simulink model "LQR_controller_V2"  (R2023b)
settings: Solver=VariableStepAuto  StartTime=0.0  StopTime=10.0  RelTol=1e-3
undefined symbols (not defined in the file): A_obs, B_obs, C_obs, K_f_lqr, K_lqr, L
libraries: cstblocks x1
settings Model: Creator=torb  LastModifiedBy=torb

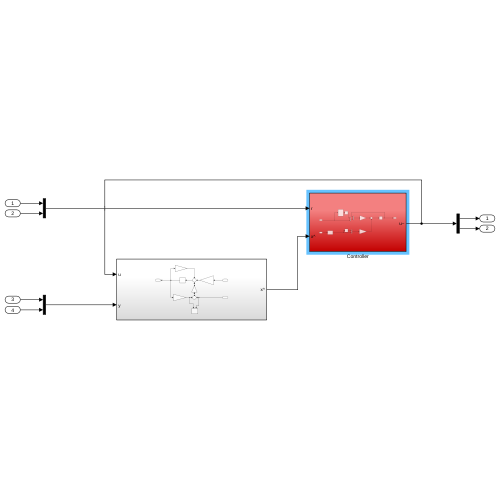
[thumbnail: Simulink's stored preview of the top-level diagram]
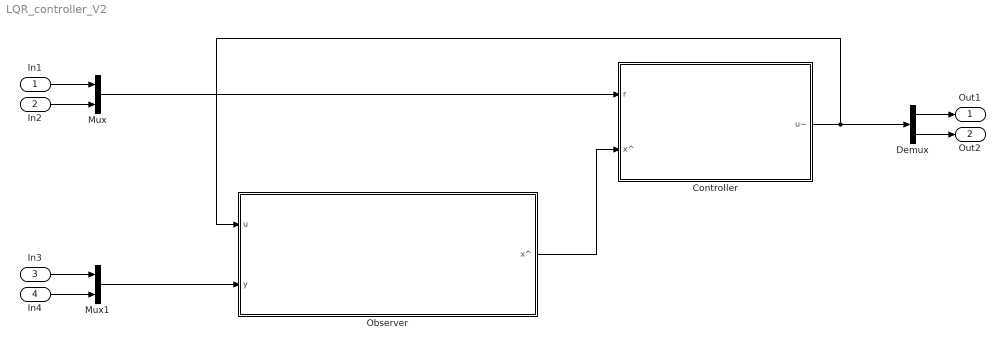
== system LQR_controller_V2 ==
  In1 : Inport
  In2 : Inport  Port=2
  In3 : Inport  Port=3
  In4 : Inport  Port=4
  Controller : Subsystem
  Demux : Demux  Outputs=2
  Mux : Mux  Inputs=2
  Mux1 : Mux  Inputs=2
  Observer : Subsystem
  Out1 : Outport
  Out2 : Outport  Port=2
  wires:
  Mux/1 -> Controller/1(r)
  Controller/1(u~) -> Demux/1, Observer/1(u)
  Observer/1(x^) -> Controller/2(x^)
  Mux1/1 -> Observer/2(y)
  In1/1 -> Mux/1
  In2/1 -> Mux/2
  In3/1 -> Mux1/1
  In4/1 -> Mux1/2
  Demux/2 -> Out2/1
  Demux/1 -> Out1/1

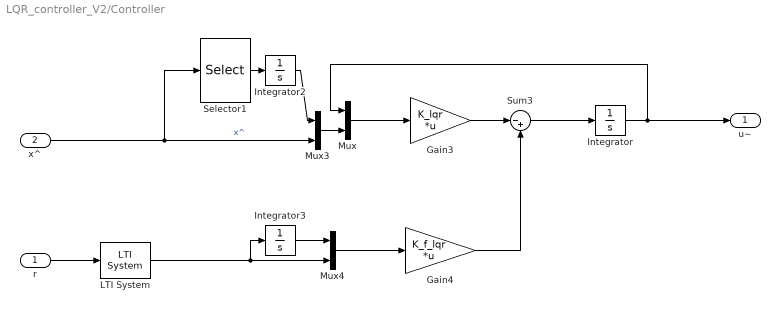
== system LQR_controller_V2/Controller ==
  r : Inport
  x^ : Inport  Port=2
  Gain3 : Gain  Gain=K_lqr  Multiplication=Matrix(K*u)
  Gain4 : Gain  Gain=K_f_lqr  Multiplication=Matrix(K*u)
  Integrator : Integrator  InitialCondition=[0;0]
  Integrator2 : Integrator
  Integrator3 : Integrator
  LTI System : cstblocks/LTI System  sys=ref_filter  IC=[]  PadeOrder=0
  Mux : Mux  Inputs=2
  Mux3 : Mux  Inputs=2
  Mux4 : Mux  Inputs=2
  Selector1 : Selector  InputPortWidth=6  IndexOptions=Index vector (dialog)  Indices=[1 2]  OutputSizes=1
  Sum3 : Sum  Inputs=|-+
  u~ : Outport
  wires:
  r/1 -> LTI System/1
  LTI System/1 -> Mux4/2, Integrator3/1
  Gain4/1 -> Sum3/2
  Gain3/1 -> Sum3/1
  Sum3/1 -> Integrator/1
  Selector1/1 -> Integrator2/1
  Integrator2/1 -> Mux3/1
  x^/1 -> Selector1/1, Mux3/2  "x^"
  Integrator3/1 -> Mux4/1
  Integrator/1 -> Mux/1, u~/1
  Mux3/1 -> Mux/2
  Mux/1 -> Gain3/1
  Mux4/1 -> Gain4/1

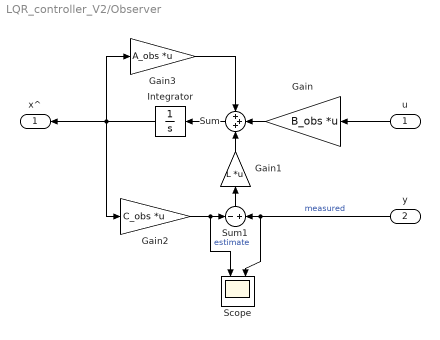
== system LQR_controller_V2/Observer ==
  u : Inport
  y : Inport  Port=2
  Gain : Gain  Gain=B_obs  Multiplication=Matrix(K*u)
  Gain1 : Gain  Gain=L  Multiplication=Matrix(K*u)
  Gain2 : Gain  Gain=C_obs  Multiplication=Matrix(K*u)
  Gain3 : Gain  Gain=A_obs  Multiplication=Matrix(K*u)
  Integrator : Integrator
  Scope : Scope  NumInputPorts=2
  Sum : Sum  Inputs=+++
  Sum1 : Sum  Inputs=-|+
  x^ : Outport
  wires:
  Gain/1 -> Sum/2
  Sum/1 -> Integrator/1
  Integrator/1 -> Gain2/1, x^/1, Gain3/1
  Gain2/1 -> Scope/1, Sum1/1  "estimate"
  Gain1/1 -> Sum/3
  Sum1/1 -> Gain1/1
  Gain3/1 -> Sum/1
  y/1 -> Scope/2, Sum1/2  "measured"
  u/1 -> Gain/1
